simulink model "shape_diff"  (R2020b)
settings: Solver=VariableStepAuto  StartTime=0.0  StopTime=10.0  RelTol=1e-3
values from neighbouring files (symbols this model uses):
  v_LED = .02    (= 0.02)    [zz_cfd.m]
  v_threshold = (1.8/(2^9)) * 71    (= 0.249609375)    [zz_noShape.m]
libraries: simulink x2
settings Model: Creator=lydialee  LastModifiedBy=lydialee
settings SFSimCC: CustomCodeUndefinedFunction=UseInterfaceOnly

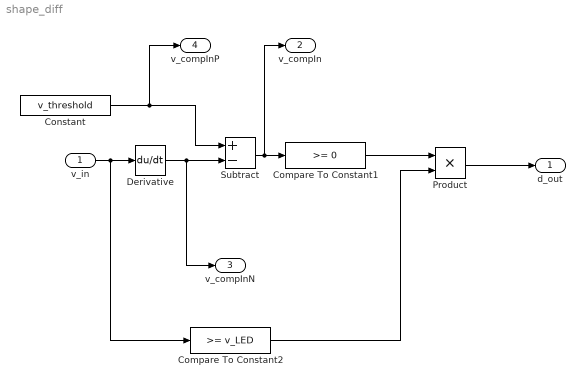
== system shape_diff ==
  v_in : Inport
  Compare To Constant1 : simulink/Logic and Bit Operations/Compare To Constant  relop=>=  const=0  OutDataTypeStr=boolean
  Compare To Constant2 : simulink/Logic and Bit Operations/Compare To Constant  relop=>=  const=v_LED  OutDataTypeStr=boolean
  Constant : Constant  Value=v_threshold
  Derivative : Derivative
  Product : Product
  Subtract : Sum  Inputs=+-
  d_out : Outport  VectorParamsAs1DForOutWhenUnconnected=off
  v_compIn : Outport  Port=2  VectorParamsAs1DForOutWhenUnconnected=off
  v_compInN : Outport  Port=3  VectorParamsAs1DForOutWhenUnconnected=off
  v_compInP : Outport  Port=4  VectorParamsAs1DForOutWhenUnconnected=off
  wires:
  Derivative/1 -> v_compInN/1, Subtract/2
  v_in/1 -> Compare To Constant2/1, Derivative/1
  Subtract/1 -> v_compIn/1, Compare To Constant1/1
  Constant/1 -> Subtract/1, v_compInP/1
  Compare To Constant1/1 -> Product/1
  Compare To Constant2/1 -> Product/2
  Product/1 -> d_out/1
